simulink model "positionSimulation"  (R2026a)
settings: Solver=VariableStepAuto
undefined symbols (not defined in the file): G_theta_x, minreal
libraries: cstblocks_lti x5
settings Model: Creator=Maria  LastModifiedBy=Maria

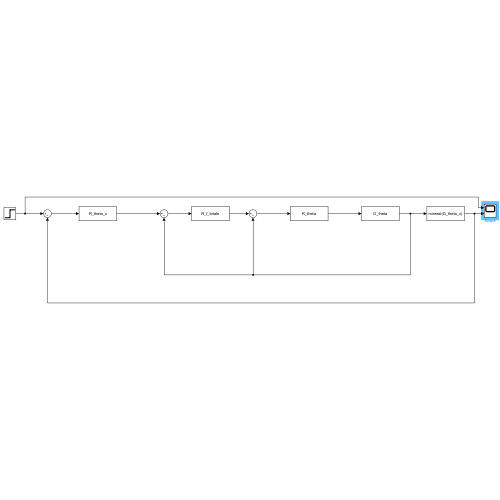
[thumbnail: Simulink's stored preview of the top-level diagram]
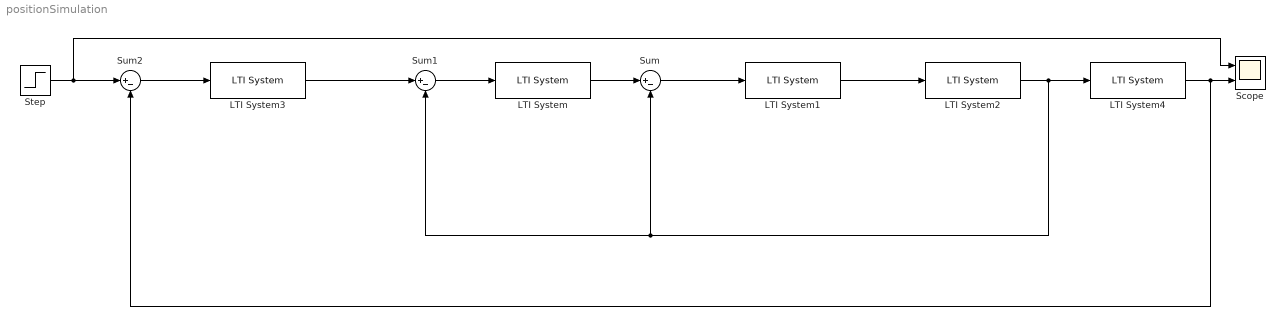
== system positionSimulation ==
  LTI System : cstblocks_lti/LTI System  sys=R_f_totale  IC=[]  PadeOrder=0
      settings: LibrarySourceBlock=cstblocks/LTI System
  LTI System1 : cstblocks_lti/LTI System  sys=R_theta  IC=[]  PadeOrder=0
      settings: LibrarySourceBlock=cstblocks/LTI System
  LTI System2 : cstblocks_lti/LTI System  sys=G_theta  IC=[]  PadeOrder=0
      settings: LibrarySourceBlock=cstblocks/LTI System
  LTI System3 : cstblocks_lti/LTI System  sys=R_theta_x  IC=[]  PadeOrder=0
      settings: LibrarySourceBlock=cstblocks/LTI System
  LTI System4 : cstblocks_lti/LTI System  sys=minreal(G_theta_x)  IC=[]  PadeOrder=0
      settings: LibrarySourceBlock=cstblocks/LTI System
  Scope : Scope  NumInputPorts=2
      settings: ActiveDisplayYMinimum=-1  ActiveDisplayYMaximum=1
  Step : Step  FinalValue=0.1  SampleTime=0
  Sum : Sum  Inputs=|+-
  Sum1 : Sum  Inputs=|+-
  Sum2 : Sum  Inputs=|+-
  wires:
  LTI System2/1 -> LTI System4/1, Sum1/2, Sum/2
  LTI System/1 -> Sum/1
  LTI System1/1 -> LTI System2/1
  Sum/1 -> LTI System1/1
  Sum1/1 -> LTI System/1
  Step/1 -> Sum2/1, Scope/1
  Sum2/1 -> LTI System3/1
  LTI System3/1 -> Sum1/1
  LTI System4/1 -> Sum2/2, Scope/2
